simulink model "q_aero_step_response_pitch_from_yaw"  (R2014a)
settings: Solver=ode1  StartTime=0.0  StopTime=5  FixedStep=0.002  RelTol=1e-3
libraries: quarc_library x2, quanser_aero x1
settings Model: SimulationMode=external  ExtModeTrigDuration=5000  Creator=MLevis  LastModifiedBy=MLevis
settings SolverCC: PositivePriorityOrder=on
settings DebuggingCC: MergeDetectMultiDrivingBlocksExec=error
settings RTWCC: SystemTargetFile=quarc_win64.tlc  TemplateMakefile=quarc_default_tmf  Description=QUARC Win64 Target  ProcessScript=quarc_win64_make_rtw_hook
settings GRTTargetCC: ParMdlRefBuildCompliant=off  CompOptLevelCompliant=off  CombineOutputUpdateFcns=off  MatFileLogging=off  CPPClassGenCompliant=off  GRTInterface=on  ExtMode=on  ExtModeMexFile=quarc_comm

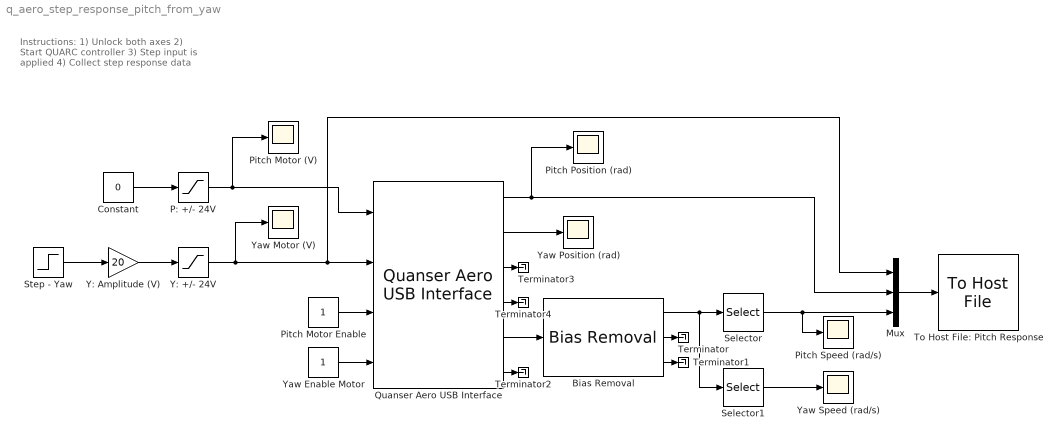
== system q_aero_step_response_pitch_from_yaw ==
  note: Instructions:
      | 1) Unlock both axes
      | 2) Start QUARC controller
      | 3) Step input is applied
      | 4) Collect step response data
  Bias Removal : quarc_library/Discrete/Bias Removal  start_time=0  end_time=1  switch_id=0  sample_time=qc_get_step_size
  Constant : Constant  Value=0
  Mux : Mux  Inputs=3
  P: +/- 24V : Saturate  UpperLimit=24  LowerLimit=-24
  Pitch Motor (V) : Scope
      settings: TimeRange=5  YMin=-25  YMax=25  SaveName=ScopeData2
  Pitch Motor Enable : Constant
  Pitch Position (rad) : Scope
      settings: TimeRange=5  YMin=-1.5  YMax=1.5  SaveName=ScopeData3
  Pitch Speed (rad/s) : Scope
      settings: TimeRange=5  YMin=-1.5  YMax=1.5  SaveName=pitch_spd
  Quanser Aero USB Interface : quanser_aero/Quanser Aero USB Interface
  Selector : Selector  InputPortWidth=3  Indices=[2]
  Selector1 : Selector  InputPortWidth=3  Indices=[3]
  Step - Yaw : Step  SampleTime=0
  Terminator{,1..4} (5 alike) : Terminator
  To Host File: Pitch Response : quarc_library/Sinks/To Host/To Host File  file_name=aero_pitch_from_yaw_step_rsp.mat  variable_name=step_rsp_py  decimation=1  sample_time=-1  file_format=MAT-file v.4  options=No header or footer  append=off  final_file_name=aero_pitch_from_yaw_step_rsp.mat
  Y: +/- 24V : Saturate  UpperLimit=24  LowerLimit=-24
  Y: Amplitude (V) : Gain  Gain=20
  Yaw Enable Motor : Constant
  Yaw Motor (V) : Scope
      settings: TimeRange=5  YMin=-25  YMax=25  SaveName=ScopeData5
  Yaw Position (rad) : Scope
      settings: TimeRange=5  YMin=-0.5  YMax=1.5  SaveName=ScopeData4
  Yaw Speed (rad/s) : Scope
      settings: TimeRange=5  YMin=-0.5  YMax=1.5  SaveName=pitch_spd1
  wires:
  Pitch Motor Enable/1 -> Quanser Aero USB Interface/3
  Yaw Enable Motor/1 -> Quanser Aero USB Interface/4
  P: +/- 24V/1 -> Quanser Aero USB Interface/1, Pitch Motor (V)/1
  Constant/1 -> P: +/- 24V/1
  Quanser Aero USB Interface/1 -> Mux/2, Pitch Position (rad)/1
  Quanser Aero USB Interface/2 -> Yaw Position (rad)/1
  Mux/1 -> To Host File: Pitch Response/1
  Bias Removal/2 -> Terminator/1
  Bias Removal/3 -> Terminator1/1
  Quanser Aero USB Interface/3 -> Terminator3/1
  Quanser Aero USB Interface/4 -> Terminator4/1
  Quanser Aero USB Interface/5 -> Bias Removal/1
  Bias Removal/1 -> Selector1/1, Selector/1
  Selector/1 -> Pitch Speed (rad/s)/1, Mux/3
  Step - Yaw/1 -> Y: Amplitude (V)/1
  Y: Amplitude (V)/1 -> Y: +/- 24V/1
  Selector1/1 -> Yaw Speed (rad/s)/1
  Y: +/- 24V/1 -> Quanser Aero USB Interface/2, Mux/1, Yaw Motor (V)/1
  Quanser Aero USB Interface/6 -> Terminator2/1
